simulink model "A2_2_Inverses_Pendel_PR"  (R2023b)
settings: Solver=FixedStepAuto  StartTime=0.0  StopTime=Te  FixedStep=Ts  RelTol=1e-3
values from neighbouring files (symbols this model uses):
  k = lqr(sys, Q, R)    [init_elast_Getriebe.m]    (also in init_inverse_pendel_pr.m)
  params = [ig c s ms CA CM]    [init_DSMS.m]    (also in init_DSMS_vorlage.m = [m c d g]; init_elast_Getriebe.m = [ig c s ms C_A_S C_M_S d]; init_inv.m = [m1 m2 l1 l2 s1 s2 C_1_S g d1 d2 m A_P B_P ig C_M]; init_inverse_pendel.m = [m1 m2 l1 l2 s1 s2 C_1_S g ig C_M_S])
  Ta = 1e-3    (= 0.001)    [init_inverse_pendel_pr.m]
  x1_ic = zeros(4,1)    [init_DSMS.m]    (also in init_DSMS_vorlage.m = zeros(2,1); init_elast_Getriebe.m; init_inv.m; init_inverse_pendel.m)
settings Model: Creator=Flo  LastModifiedBy=Flo

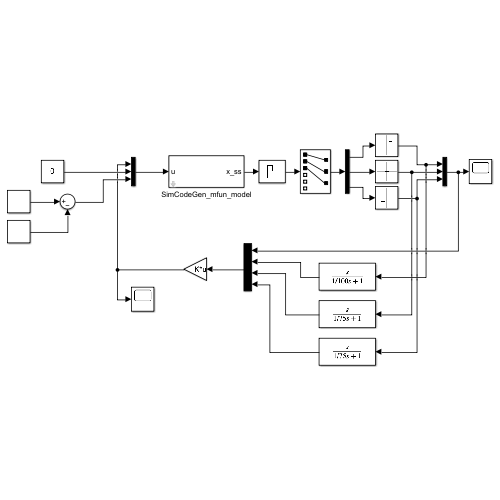
[thumbnail: Simulink's stored preview of the top-level diagram]
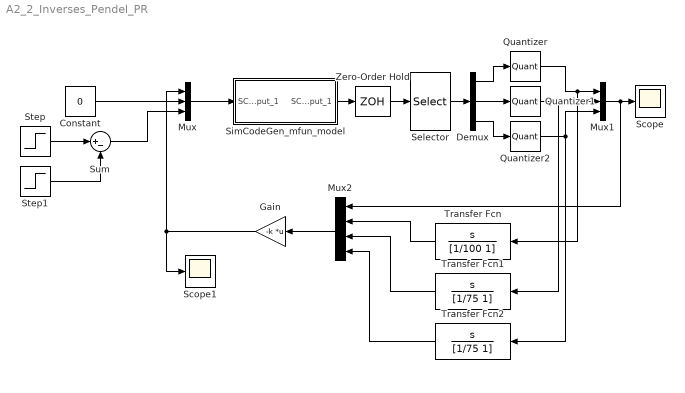
== system A2_2_Inverses_Pendel_PR ==
  Constant : Constant  Value=0
  Demux : Demux  Outputs=3
  Gain : Gain  Gain=-k  Multiplication=Matrix(K*u)
  Mux : Mux  Inputs=3
  Mux1 : Mux  Inputs=3
  Mux2 : Mux
  Quantizer : Quantizer  QuantizationInterval=2*pi/(2048*params(12))
  Quantizer1 : Quantizer  QuantizationInterval=2*pi/4096
  Quantizer2 : Quantizer  QuantizationInterval=2*pi/4096
  Scope : Scope
  Scope1 : Scope
  Selector : Selector  InputPortWidth=6  IndexOptions=Index vector (dialog)  Indices=[1 2 3]  OutputSizes=1
  SimCodeGen_mfun_model : Subsystem  mask{SC_param_0=params, SC_x1_ic=x1_ic}
      mask prompts: SC_param_0 "params"
      mask Display:
      | port_label('input', 1, 'u');
      | port_label('output', 1, 'x_ss');
  Step : Step  SampleTime=0
  Step1 : Step  Time=1.01  SampleTime=0
  Sum : Sum  Inputs=|+-
  Transfer Fcn : TransferFcn  Numerator=[1 0]  Denominator=[1/100 1]
  Transfer Fcn1 : TransferFcn  Numerator=[1 0]  Denominator=[1/75 1]
  Transfer Fcn2 : TransferFcn  Numerator=[1 0]  Denominator=[1/75 1]
  Zero-Order Hold : ZeroOrderHold  SampleTime=Ta
  wires:
  Step/1 -> Sum/1
  Step1/1 -> Sum/2
  Sum/1 -> Mux/3
  Constant/1 -> Mux/2
  Mux/1 -> SimCodeGen_mfun_model/1(SC_input_1)
  SimCodeGen_mfun_model/1(SC_output_1) -> Zero-Order Hold/1
  Gain/1 -> Scope1/1, Mux/1
  Zero-Order Hold/1 -> Selector/1
  Selector/1 -> Demux/1
  Demux/1 -> Quantizer/1
  Demux/2 -> Quantizer1/1
  Demux/3 -> Quantizer2/1
  Mux1/1 -> Mux2/1, Scope/1
  Quantizer2/1 -> Mux1/3, Transfer Fcn2/1
  Quantizer1/1 -> Transfer Fcn1/1, Mux1/2
  Quantizer/1 -> Transfer Fcn/1, Mux1/1
  Mux2/1 -> Gain/1
  Transfer Fcn/1 -> Mux2/2
  Transfer Fcn1/1 -> Mux2/3
  Transfer Fcn2/1 -> Mux2/4

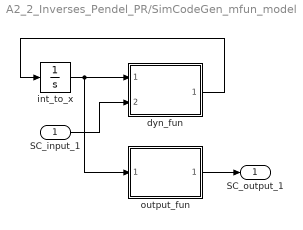
== system A2_2_Inverses_Pendel_PR/SimCodeGen_mfun_model ==
  SC_input_1 : Inport
  dyn_fun : MATLAB Function  TreatAsAtomicUnit=on
  int_to_x : Integrator  InitialCondition=[SC_x1_ic]
  output_fun : MATLAB Function  TreatAsAtomicUnit=on
  SC_output_1 : Outport
  wires:
  int_to_x/1 -> output_fun/1(SC_state), dyn_fun/1(SC_state)
  SC_input_1/1 -> dyn_fun/2(SC_input_0)
  output_fun/1(SC_output_0) -> SC_output_1/1
  dyn_fun/1(SC_state_dot) -> int_to_x/1

== matlab function A2_2_Inverses_Pendel_PR/SimCodeGen_mfun_model/dyn_fun ==
  data: SC_state input size=[6]; SC_state_dot output size=[6]; SC_input_0 input size=[3]; SC_param_0 parameter
function SC_state_dot  = dyn_fun(SC_state, SC_input_0, SC_param_0)
    SC_state_dot = zeros(6, 1);
    SC_state_x_0 = SC_state(1:6);
    SC_eval = zeros(6,1);
    SC_eval(1) = SC_state_x_0(4);
    SC_eval(2) = SC_state_x_0(5);
    SC_eval(3) = SC_state_x_0(6);
    t1 = SC_state_x_0(3);
    t2 = cos(t1);
    t3 = t2 ^ 2;
    t4 = SC_param_0(5);
    t5 = t4 ^ 2;
    t6 = t5 * t3;
    t7 = SC_param_0(6);
    t8 = t7 ^ 2;
    t9 = SC_param_0(18);
    t10 = t9 ^ 2;
    t11 = t10 * t8;
    t12 = t11 * t6;
    t15 = SC_param_0(3);
    t16 = t9 * t15;
    t17 = SC_param_0(9);
    t18 = t17 * t16;
    t21 = t15 ^ 2;
    t22 = t17 ^ 2;
    t23 = t22 * t21;
    t24 = t23 * t6;
    t26 = t8 * t5;
    t27 = SC_param_0(2);
    t28 = t9 * t27;
    t29 = t28 * t26;
    t30 = t16 * t26;
    t32 = SC_param_0(17);
    t33 = t9 * t32;
    t34 = t33 * t26;
    t36 = t10 * t26;
    t38 = t27 * t5;
    t39 = t22 * t15;
    t40 = t39 * t38;
    t41 = t21 * t5;
    t42 = t22 * t41;
    t44 = t15 * t5;
    t45 = t22 * t32;
    t46 = t45 * t44;
    t48 = t22 * t9;
    t49 = t48 * t44;
    t51 = t27 * t8;
    t52 = SC_param_0(8);
    t53 = t52 ^ 2;
    t54 = t53 * t9;
    t55 = t54 * t51;
    t57 = t15 * t27;
    t58 = t22 * t53;
    t59 = t58 * t57;
    t61 = SC_param_0(19);
    t62 = t5 * t61;
    t47 = t32 * t62;
    t73 = -0.24e2 * t18 * t6 * t7 + 0.12e2 * t27 * t53 * t61 + 0.12e2 * t15 * t62 + t27 * t62 + 0.12e2 * t62 * t9 - 0.12e2 * t12 - 0.12e2 * t24 + t29 + 0.12e2 * t30 + 0.12e2 * t34 + 0.12e2 * t36 + t40 + 0.12e2 * t42 + 0.12e2 * t46 + 0.12e2 * t47 + 0.12e2 * t49 + 0.12e2 * t55 + 0.12e2 * t59;
    t74 = SC_state_x_0(2);
    t75 = sin(t74);
    t76 = t75 * t61;
    t77 = sin(t1);
    t78 = cos(t74);
    t79 = t78 * t77;
    t80 = t79 * t76;
    t81 = t5 * t4;
    t82 = t15 * t81;
    t83 = t17 * t9;
    t84 = t83 * t82;
    t87 = t75 ^ 2;
    t88 = t87 * t61;
    t89 = t2 * t4;
    t90 = t89 * t88;
    t92 = t17 * t53 * t57;
    t95 = t5 * t2;
    t96 = t23 * t95;
    t99 = t27 * t81;
    t100 = t17 * t15;
    t101 = t100 * t99;
    t104 = t17 * t32;
    t105 = t104 * t82;
    t108 = t77 * t75;
    t109 = t2 * t78;
    t110 = t109 * t108;
    t111 = t22 ^ 2;
    t116 = t81 * t78;
    t117 = t116 * t108;
    t118 = t15 * t8;
    t119 = t17 * t10;
    t120 = t119 * t118;
    t123 = t2 * t87;
    t124 = t8 * t81;
    t125 = t124 * t123;
    t126 = t83 * t57;
    t129 = SC_param_0(4);
    t130 = t129 ^ 2;
    t131 = t130 * t3;
    t132 = t7 * t5;
    t133 = t132 * t131;
    t136 = t87 * t130;
    t137 = t77 ^ 2;
    t139 = t5 * t137 * t136;
    t140 = t15 * t7;
    t141 = t119 * t140;
    t144 = t21 * t7;
    t145 = t83 * t144;
    t148 = t78 ^ 2;
    t149 = t148 * t130;
    t150 = t6 * t149;
    t91 = t110 * t111;
    t155 = 0.24e2 * t32 * t41 * t91 + 0.2e1 * t101 * t80 + 0.24e2 * t105 * t80 + 0.24e2 * t117 * t120 + 0.2e1 * t125 * t126 - 0.24e2 * t126 * t133 - 0.24e2 * t139 * t141 - 0.24e2 * t139 * t145 + 0.24e2 * t141 * t150 + 0.24e2 * t145 * t150 + 0.24e2 * t80 * t84 + 0.24e2 * t80 * t96 + 0.24e2 * t90 * t92;
    t156 = t3 * t148;
    t157 = t26 * t156;
    t158 = t48 * t57;
    t161 = t7 * t81;
    t162 = t161 * t123;
    t165 = t21 * t8;
    t166 = t83 * t165;
    t169 = t48 * t144;
    t172 = SC_param_0(1);
    t176 = SC_param_0(7) ^ 2;
    t182 = t58 * t16;
    t185 = t27 * t4;
    t186 = t185 * t149;
    t187 = t22 * t52;
    t191 = t3 * t87;
    t192 = t5 ^ 2;
    t195 = t32 * t15;
    t196 = t83 * t195;
    t201 = t21 * t27;
    t206 = t111 * t21;
    t210 = t4 * t130;
    t211 = t210 * t156;
    t212 = t187 * t201;
    t215 = t4 * t78;
    t216 = t215 * t108;
    t217 = t22 * t17;
    t219 = t217 * t53 * t201;
    t197 = t192 * t191;
    t222 = -0.24e2 * t16 * t17 * t172 * t176 * t6 * t7 + 0.24e2 * t110 * t111 * t201 * t53 + 0.2e1 * t110 * t206 * t38 - 0.48e2 * t156 * t182 * t51 - 0.24e2 * t16 * t186 * t187 - 0.24e2 * t196 * t197 * t7 + 0.24e2 * t117 * t166 + 0.24e2 * t117 * t169 - 0.24e2 * t133 * t196 - 0.4e1 * t157 * t158 + 0.2e1 * t158 * t162 + 0.24e2 * t211 * t212 + 0.24e2 * t216 * t219;
    t227 = t27 * t7;
    t228 = t227 * t54;
    t231 = t33 * t161;
    t234 = t16 * t161;
    t237 = t11 * t95;
    t240 = t28 * t161;
    t243 = SC_param_0(13);
    t244 = SC_param_0(12);
    t245 = t244 ^ 2;
    t246 = t245 * t243;
    t247 = t5 * t246;
    t248 = t22 * t57;
    t250 = t3 * t243;
    t251 = t245 * t250;
    t255 = t53 * t15;
    t256 = t22 * t255;
    t259 = t148 * t61;
    t261 = t53 * t28;
    t264 = t3 * t61;
    t268 = t5 * t259;
    t269 = t32 * t8;
    t270 = t9 * t269;
    t273 = t5 * t264;
    t276 = -0.24e2 * t186 * t187 * t195 + 0.12e2 * t246 * t256 * t27 + 0.12e2 * t259 * t261 * t8 + 0.12e2 * t261 * t264 * t8 + 0.24e2 * t228 * t90 + 0.24e2 * t231 * t80 + 0.24e2 * t234 * t80 + 0.24e2 * t237 * t80 + 0.2e1 * t240 * t80 + t247 * t248 - 0.12e2 * t251 * t42 + 0.12e2 * t268 * t270 + 0.12e2 * t270 * t273;
    t277 = t5 * t88;
    t278 = t53 * t57;
    t283 = t3 * t259;
    t286 = t2 * t88;
    t287 = t21 * t81;
    t288 = t17 * t287;
    t297 = t130 * t259;
    t298 = t32 * t44;
    t301 = t75 * t130;
    t303 = t2 * t79 * t301;
    t304 = t15 * t227;
    t305 = t17 * t54;
    t315 = t22 * t54;
    t316 = t315 * t57;
    t325 = t305 * t57;
    t292 = t132 * t18;
    t328 = 0.48e2 * t110 * t316 * t8 + 0.24e2 * t216 * t316 * t7 + 0.24e2 * t216 * t325 * t8 + 0.12e2 * t256 * t259 * t27 + 0.12e2 * t256 * t264 * t27 + 0.4e1 * t27 * t292 * t303 + 0.48e2 * t303 * t304 * t305 + t248 * t268 + t248 * t273 + 0.24e2 * t277 * t278 - 0.24e2 * t283 * t42 + 0.24e2 * t286 * t288 - 0.24e2 * t297 * t298;
    t333 = t52 * t9;
    t334 = t17 * t333;
    t338 = t8 * t4;
    t339 = t10 * t27;
    t351 = t48 * t195;
    t356 = t338 * t149;
    t357 = t32 * t27;
    t365 = t52 * t10 * t51;
    t368 = t8 * t7;
    t369 = t27 * t368;
    t370 = t53 * t10;
    t371 = t370 * t369;
    t374 = t8 ^ 2;
    t375 = t27 * t374;
    t379 = t5 * t245;
    t381 = t83 * t140;
    t384 = t374 * t5;
    t385 = t10 * t32;
    t389 = 0.48e2 * t334 * t57 * t7 * t210 * t156 - 0.24e2 * t52 * t339 * t338 * t303 - 0.24e2 * t21 * t185 * t303 * t187 + 0.24e2 * t196 * t125 + 0.24e2 * t351 * t162 - 0.48e2 * t351 * t157 - 0.24e2 * t333 * t357 * t356 - 0.24e2 * t333 * t57 * t356 + 0.24e2 * t365 * t211 + 0.24e2 * t371 * t216 + 0.24e2 * t370 * t375 * t110 - 0.24e2 * t381 * t379 * t250 + 0.24e2 * t385 * t384 * t110;
    t393 = t10 * t15;
    t401 = t22 * t10;
    t402 = t401 * t140;
    t405 = t5 * t109;
    t406 = t405 * t108;
    t407 = t22 * t33;
    t411 = t22 * t16;
    t415 = t79 * t301;
    t416 = t22 * t201;
    t420 = t27 * t2;
    t421 = t53 * t21;
    t422 = t22 * t421;
    t426 = t10 * t51;
    t430 = t8 * t2;
    t431 = t53 * t339;
    t435 = t22 * t393;
    t436 = t435 * t26;
    t439 = t3 * t2;
    t441 = t439 * t78 * t108;
    t444 = t3 * t78;
    t445 = t444 * t108;
    t446 = t17 * t393;
    t450 = 0.2e1 * t110 * t339 * t384 + 0.24e2 * t110 * t384 * t393 + 0.48e2 * t118 * t406 * t407 - 0.72e2 * t124 * t445 * t446 + 0.4e1 * t406 * t411 * t51 + 0.24e2 * t41 * t9 * t91 + 0.2e1 * t415 * t416 * t95 + 0.24e2 * t415 * t420 * t422 + 0.2e1 * t415 * t426 * t95 + 0.24e2 * t415 * t430 * t431 + 0.48e2 * t110 * t436 + 0.24e2 * t117 * t402 - 0.24e2 * t436 * t441;
    t452 = t9 * t21;
    t453 = t22 * t452;
    t454 = t453 * t26;
    t464 = t217 * t452;
    t476 = t18 * t227;
    t484 = t7 * t4;
    t437 = t3 * t149;
    t438 = t325 * t7;
    t495 = -0.48e2 * t368 * t441 * t446 * t5 + 0.2e1 * t117 * t18 * t51 + 0.2e1 * t117 * t227 * t411 + 0.24e2 * t123 * t316 * t484 + 0.24e2 * t123 * t325 * t338 - 0.24e2 * t132 * t191 * t325 - 0.48e2 * t132 * t441 * t464 - 0.72e2 * t161 * t445 * t453 + 0.48e2 * t110 * t454 - 0.2e1 * t139 * t476 - 0.2e1 * t150 * t476 - 0.24e2 * t437 * t438 - 0.24e2 * t441 * t454;
    t500 = t17 * t33;
    t507 = t500 * t140;
    t515 = t17 * t255;
    t522 = t22 * t195;
    t526 = t9 * t51;
    t530 = t9 * t118;
    t486 = t137 * t136;
    t543 = 0.24e2 * t117 * t118 * t500 + 0.24e2 * t117 * t140 * t407 + 0.24e2 * t185 * t515 * t80 + 0.2e1 * t248 * t80 * t95 + 0.24e2 * t256 * t420 * t80 + 0.24e2 * t261 * t430 * t80 + 0.24e2 * t261 * t484 * t80 + 0.24e2 * t411 * t80 * t95 + 0.24e2 * t522 * t80 * t95 + 0.2e1 * t526 * t80 * t95 + 0.24e2 * t530 * t80 * t95 - 0.24e2 * t139 * t507 + 0.24e2 * t150 * t507 - 0.24e2 * t438 * t486;
    t550 = SC_param_0(10);
    t551 = t550 * t61;
    t552 = t9 * t5;
    t558 = t130 * t61;
    t559 = t10 * t5;
    t562 = t32 * t5;
    t565 = t32 ^ 2;
    t569 = t565 * t5;
    t572 = t27 * t53;
    t578 = t27 ^ 2;
    t579 = t53 * t578;
    t582 = t53 ^ 2;
    t588 = 0.12e2 * t10 * t192 * t88 + 0.12e2 * t192 * t565 * t88 + 0.24e2 * t270 * t80 * t95 + 0.12e2 * t578 * t582 * t88 + t38 * t551 + 0.12e2 * t41 * t558 + 0.12e2 * t44 * t551 + 0.12e2 * t551 * t552 + 0.12e2 * t551 * t562 + 0.12e2 * t551 * t572 + 0.12e2 * t558 * t559 + 0.12e2 * t558 * t569 + 0.12e2 * t558 * t579;
    t589 = t578 * t5;
    t594 = t5 * t550;
    t597 = t192 * t87;
    t598 = t10 * t9;
    t599 = t598 * t8;
    t602 = t5 * t148;
    t603 = t598 * t374;
    t608 = t3 ^ 2;
    t609 = t5 * t608;
    t612 = t5 * t130;
    t617 = t21 * t15;
    t618 = t22 * t617;
    t621 = t111 * t617;
    t628 = 0.12e2 * t192 * t21 * t88 + 0.12e2 * t11 * t594 + 0.12e2 * t23 * t594 + t558 * t589 + 0.12e2 * t597 * t599 + 0.12e2 * t597 * t618 + 0.12e2 * t599 * t612 + 0.12e2 * t6 * t603 + 0.12e2 * t602 * t603 + 0.12e2 * t602 * t621 - 0.12e2 * t603 * t609 - 0.12e2 * t609 * t621 + 0.12e2 * t612 * t618;
    t632 = t78 * t108;
    t633 = t130 * t2;
    t634 = t4 * t633;
    t639 = t8 * t602;
    t642 = t8 * t6;
    t645 = t5 * t87;
    t646 = t27 * t645;
    t650 = t486;
    t651 = t45 * t41;
    t654 = t437;
    t661 = t58 * t201;
    t666 = t4 * t149;
    t669 = t4 * t123;
    t672 = t5 * t191;
    t675 = 0.24e2 * t217 * t287 * t32 * t632 - 0.48e2 * t304 * t334 * t632 * t634 + 0.24e2 * t195 * t58 * t646 + 0.2e1 * t158 * t639 + 0.2e1 * t158 * t642 - 0.24e2 * t212 * t666 + 0.24e2 * t219 * t669 + 0.12e2 * t6 * t621 - 0.12e2 * t650 * t651 - 0.12e2 * t650 * t661 + 0.12e2 * t651 * t654 - 0.12e2 * t654 * t661 - 0.12e2 * t661 * t672;
    t676 = t23 * t38;
    t679 = t217 * t21;
    t691 = t5 * t439;
    t695 = t5 * t156;
    t696 = t15 * t368;
    t697 = t119 * t696;
    t700 = t217 * t9;
    t701 = t700 * t144;
    t704 = t393 * t26;
    t709 = t368 * t81;
    t713 = t339 * t26;
    t657 = t217 * t617;
    t658 = t632 * t81 * t3;
    t670 = t632 * t621;
    t719 = 0.2e1 * t339 * t632 * t709 + 0.24e2 * t393 * t632 * t709 + 0.2e1 * t632 * t679 * t99 - t650 * t676 - 0.12e2 * t650 * t704 - t650 * t713 - t654 * t676 + 0.12e2 * t654 * t704 - t654 * t713 - 0.24e2 * t657 * t658 - 0.24e2 * t670 * t691 + 0.24e2 * t670 * t95 - 0.24e2 * t695 * t697 - 0.24e2 * t695 * t701;
    t732 = t8 * t645;
    t736 = t5 * t149;
    t743 = t385 * t26;
    t754 = t3 * t550;
    t758 = t370 * t51;
    t720 = t632 * t603;
    t761 = -0.24e2 * t118 * t33 * t736 + 0.24e2 * t357 * t54 * t732 - 0.24e2 * t368 * t598 * t658 - 0.24e2 * t381 * t5 * t754 + 0.24e2 * t385 * t632 * t709 + 0.24e2 * t351 * t639 + 0.24e2 * t351 * t642 - 0.24e2 * t351 * t736 - 0.12e2 * t650 * t743 + 0.12e2 * t654 * t743 - 0.12e2 * t654 * t758 - 0.24e2 * t691 * t720 + 0.24e2 * t720 * t95;
    t775 = t8 * t148;
    t779 = t8 * t3;
    t783 = t48 * t41;
    t791 = t5 * t131;
    t739 = t27 * t182;
    t796 = 0.24e2 * t287 * t632 * t700 + 0.24e2 * t54 * t57 * t732 - 0.24e2 * t141 * t791 - 0.24e2 * t145 * t791 + 0.24e2 * t182 * t646 - 0.24e2 * t365 * t666 + 0.24e2 * t371 * t669 - 0.12e2 * t650 * t758 - 0.12e2 * t650 * t783 + 0.12e2 * t654 * t783 - 0.12e2 * t672 * t758 + 0.24e2 * t739 * t775 + 0.24e2 * t739 * t779;
    t798 = t77 * t76;
    t799 = t10 * t7;
    t772 = t185 * t297;
    t777 = t798 * t116;
    t830 = -0.24e2 * t32 * t52 * t772 + 0.24e2 * t231 * t286 + 0.24e2 * t234 * t286 + 0.2e1 * t240 * t286 - 0.2e1 * t283 * t29 - 0.24e2 * t283 * t30 - 0.24e2 * t283 * t34 - 0.24e2 * t283 * t46 - 0.24e2 * t283 * t49 - 0.24e2 * t283 * t55 + 0.24e2 * t286 * t84 - 0.24e2 * t333 * t772 + 0.24e2 * t777 * t799;
    t833 = t52 * t15;
    t839 = t17 * t21;
    t847 = t48 * t165;
    t850 = t81 * t123;
    t853 = t401 * t118;
    t858 = t608 * t148;
    t859 = t5 * t858;
    t862 = t439 * t87;
    t863 = t81 * t862;
    t870 = 0.2e1 * t101 * t286 + 0.24e2 * t105 * t286 + 0.24e2 * t120 * t850 - 0.72e2 * t120 * t863 + 0.24e2 * t166 * t850 - 0.2e1 * t283 * t40 - 0.24e2 * t283 * t59 + 0.24e2 * t402 * t850 - 0.60e2 * t695 * t847 - 0.60e2 * t695 * t853 - 0.24e2 * t772 * t833 + 0.24e2 * t777 * t839 + 0.24e2 * t847 * t859 + 0.24e2 * t853 * t859;
    t883 = t197;
    t889 = t10 * t32 * t374;
    t895 = t9 * t565 * t8;
    t898 = t10 * t269;
    t904 = t176 * t10 * t172;
    t907 = t8 * t130;
    t908 = t9 * t578;
    t909 = t53 * t908;
    t912 = -0.24e2 * t141 * t883 - 0.24e2 * t145 * t883 + 0.24e2 * t169 * t850 - 0.72e2 * t169 * t863 + 0.12e2 * t26 * t904 + 0.12e2 * t270 * t594 + 0.12e2 * t6 * t889 + 0.12e2 * t602 * t889 + 0.12e2 * t612 * t895 + 0.24e2 * t612 * t898 + 0.48e2 * t697 * t859 + 0.48e2 * t701 * t859 + 0.12e2 * t907 * t909;
    t915 = t8 * t87;
    t919 = t374 * t148;
    t922 = t374 * t3;
    t933 = t111 * t452;
    t943 = 0.12e2 * t582 * t908 * t915 - 0.12e2 * t36 * t754 + 0.12e2 * t431 * t907 + 0.12e2 * t431 * t919 + 0.12e2 * t431 * t922 + 0.12e2 * t435 * t597 + 0.12e2 * t435 * t612 + 0.24e2 * t453 * t597 + 0.24e2 * t453 * t612 + t526 * t594 + 0.12e2 * t530 * t594 + 0.12e2 * t6 * t933 + 0.12e2 * t602 * t933;
    t945 = t8 * t550;
    t952 = t598 * t384;
    t955 = t598 * t709;
    t966 = t9 * t165;
    t969 = t10 * t118;
    t977 = t598 * t26;
    t913 = t578 * t612;
    t914 = t8 * t9;
    t980 = 0.24e2 * t123 * t955 - 0.12e2 * t131 * t977 - 0.36e2 * t156 * t952 + 0.12e2 * t246 * t36 + 0.12e2 * t261 * t945 + 0.12e2 * t411 * t594 + 0.13e2 * t426 * t612 - 0.12e2 * t599 * t883 + 0.12e2 * t612 * t966 + 0.24e2 * t612 * t969 + 0.24e2 * t858 * t952 - 0.24e2 * t862 * t955 + t913 * t914;
    t988 = t10 * t15 * t374;
    t994 = t10 * t375;
    t1001 = t32 * t21;
    t1002 = t22 * t1001;
    t1006 = t22 * t565 * t15;
    t1011 = 0.24e2 * t1002 * t597 + 0.24e2 * t1002 * t612 + 0.12e2 * t1006 * t612 - 0.12e2 * t149 * t977 + t426 * t597 + 0.12e2 * t597 * t895 + 0.24e2 * t597 * t898 + 0.12e2 * t597 * t966 + 0.24e2 * t597 * t969 + 0.12e2 * t6 * t988 + t6 * t994 + 0.12e2 * t602 * t988 + t602 * t994;
    t1016 = t111 * t1001;
    t1024 = t176 * t9 * t172;
    t1029 = t243 * t61;
    t1033 = t21 * t612;
    t1042 = t10 * t612;
    t1045 = t9 * t44;
    t1048 = t15 * t192;
    t1052 = 0.12e2 * t1029 * t379 * t9 + 0.24e2 * t1048 * t88 * t9 + 0.13e2 * t15 * t38 * t558 + 0.13e2 * t38 * t558 * t9 + 0.12e2 * t1006 * t597 + 0.12e2 * t1016 * t6 + 0.12e2 * t1016 * t602 + 0.12e2 * t1024 * t62 - 0.12e2 * t1033 * t259 - 0.12e2 * t1042 * t259 + 0.24e2 * t1045 * t558 + 0.12e2 * t261 * t558 + 0.12e2 * t522 * t594;
    t1053 = t27 * t192;
    t1064 = t9 * t562;
    t1072 = t565 * t612;
    t1086 = t53 * t357;
    t1089 = 0.24e2 * t192 * t32 * t88 * t9 + 0.24e2 * t1048 * t32 * t88 + t1053 * t15 * t88 + t1053 * t32 * t88 + t1053 * t88 * t9 + 0.12e2 * t172 * t176 * t47 + 0.13e2 * t32 * t38 * t558 + 0.24e2 * t1064 * t558 - 0.12e2 * t1072 * t259 + 0.12e2 * t1086 * t558 + 0.12e2 * t259 * t36 + 0.12e2 * t264 * t36 + 0.24e2 * t298 * t558;
    t1094 = t15 * t172;
    t1098 = t27 * t172;
    t1101 = t578 * t130;
    t1102 = t53 * t1101;
    t1109 = t172 * t61;
    t1110 = t176 * t27;
    t1127 = t617 * t5;
    t1128 = t22 * t1127;
    t1050 = t245 * t1029;
    t1131 = 0.12e2 * t1029 * t15 * t379 + t1029 * t27 * t379 + 0.12e2 * t1029 * t32 * t379 + 0.12e2 * t1094 * t176 * t62 + t1098 * t176 * t62 + 0.12e2 * t1109 * t1110 * t53 + t53 * t589 * t88 + 0.12e2 * t1050 * t572 - 0.12e2 * t1102 * t259 - 0.12e2 * t1128 * t131 + 0.12e2 * t259 * t42 + 0.12e2 * t264 * t42 + 0.12e2 * t278 * t558;
    t1140 = t111 * t201;
    t1154 = t81 * t657;
    t1085 = t176 * t22;
    t1159 = t21 * t1085;
    t1162 = t172 * t5;
    t1164 = t176 * t15;
    t1087 = t1162 * t1164;
    t1170 = t1087 * t22 * t27 - 0.12e2 * t1159 * t172 * t6 - 0.12e2 * t149 * t256 * t578 + 0.2e1 * t201 * t217 * t850 - 0.12e2 * t1128 * t149 - 0.12e2 * t1128 * t650 + 0.12e2 * t1128 * t654 + t1140 * t602 - 0.2e1 * t1140 * t695 + 0.24e2 * t1154 * t632 + t39 * t913 + t416 * t597 + 0.13e2 * t416 * t612 - 0.12e2 * t416 * t791;
    t1183 = t27 * t156;
    t1184 = t111 * t421;
    t1123 = t1098 * t53 * t176;
    t1203 = t256 * t578 * t645 - 0.24e2 * t1045 * t297 - 0.24e2 * t1064 * t297 + 0.24e2 * t1086 * t277 + 0.12e2 * t1123 * t39 - 0.24e2 * t1183 * t1184 + 0.12e2 * t268 * t411 + 0.12e2 * t268 * t522 + t268 * t526 + 0.12e2 * t273 * t411 + 0.12e2 * t273 * t522 + t273 * t526 + 0.24e2 * t422 * t646;
    t1206 = t10 * t161;
    t1228 = t8 * t612;
    t1229 = t9 * t57;
    t1234 = 0.2e1 * t10 * t369 * t850 + 0.24e2 * t1206 * t286 + 0.13e2 * t1228 * t1229 + 0.12e2 * t247 * t270 + 0.24e2 * t261 * t277 + 0.12e2 * t268 * t530 + 0.12e2 * t273 * t530 - 0.24e2 * t283 * t36 - 0.12e2 * t426 * t791 - 0.12e2 * t650 * t977 + 0.12e2 * t654 * t977 - 0.2e1 * t695 * t994 - 0.12e2 * t736 * t966;
    t1242 = t8 * t597;
    t1253 = t172 * t26;
    t1265 = t27 * t907;
    t1193 = t176 * t1253;
    t1269 = 0.24e2 * t10 * t696 * t850 + 0.12e2 * t1253 * t16 * t176 + 0.12e2 * t1265 * t16 * t53 - 0.12e2 * t149 * t8 * t909 - 0.24e2 * t156 * t374 * t431 + t1193 * t28 + t1229 * t1242 + 0.24e2 * t632 * t955 - 0.12e2 * t642 * t904 - 0.24e2 * t695 * t988 - 0.24e2 * t736 * t969 - 0.12e2 * t791 * t969 - 0.12e2 * t883 * t969;
    t1275 = t176 * t9;
    t1279 = t27 * t612;
    t1296 = t9 * t195;
    t1222 = t1275 * t172 * t8;
    t1232 = t407 * t15;
    t1308 = 0.12e2 * t1265 * t33 * t53 + 0.24e2 * t368 * t385 * t850 + 0.12e2 * t1193 * t33 + 0.12e2 * t1222 * t572 + 0.24e2 * t1232 * t612 + 0.24e2 * t1242 * t1296 + 0.13e2 * t1279 * t411 + 0.24e2 * t431 * t732 - 0.12e2 * t435 * t736 - 0.24e2 * t453 * t736 - 0.12e2 * t453 * t791 - 0.24e2 * t695 * t889 + t732 * t909 - 0.12e2 * t883 * t898;
    t1311 = t9 * t357;
    t1330 = t27 * t597;
    t1339 = 0.24e2 * t1001 * t217 * t850 - 0.24e2 * t1002 * t736 - 0.12e2 * t1002 * t791 - 0.12e2 * t1002 * t883 - 0.12e2 * t1006 * t736 - 0.24e2 * t1016 * t695 + 0.24e2 * t1228 * t1296 + 0.13e2 * t1228 * t1311 + 0.13e2 * t1279 * t522 + t1330 * t522 - 0.12e2 * t736 * t895 - 0.24e2 * t736 * t898 - 0.12e2 * t791 * t898;
    t1340 = t15 * t1162;
    t1341 = t176 * t32;
    t1345 = t27 * t130;
    t1346 = t15 * t1345;
    t1347 = t53 * t32;
    t1375 = 0.12e2 * t1340 * t1341 * t22 + 0.12e2 * t1346 * t1347 * t22 - 0.24e2 * t368 * t446 * t609 - 0.24e2 * t464 * t609 * t7 + 0.24e2 * t1232 * t597 + t1330 * t411 + 0.12e2 * t247 * t522 + 0.24e2 * t435 * t639 + 0.24e2 * t453 * t639 + 0.24e2 * t453 * t642 - 0.12e2 * t453 * t883 + 0.24e2 * t464 * t850 - 0.24e2 * t695 * t933;
    t1379 = t8 * t609;
    t1401 = t111 * t1127;
    t1404 = 0.12e2 * t1275 * t1340 * t22 + 0.12e2 * t246 * t261 * t8 + t1140 * t6 + t1242 * t1311 + 0.12e2 * t1346 * t315 - 0.12e2 * t1379 * t435 - 0.12e2 * t1379 * t453 + 0.24e2 * t1401 * t858 + 0.12e2 * t247 * t411 + t247 * t526 + 0.12e2 * t247 * t530 - 0.12e2 * t251 * t36 + 0.24e2 * t435 * t642;
    t1421 = t578 * t87;
    t1426 = t27 * t148;
    t1429 = t27 * t3;
    t1435 = t27 * t550;
    t1440 = 0.12e2 * t1421 * t15 * t22 * t582 + 0.12e2 * t1101 * t256 + 0.24e2 * t1154 * t123 - 0.24e2 * t1154 * t862 + 0.12e2 * t1159 * t1162 + 0.12e2 * t1184 * t1426 + 0.12e2 * t1184 * t1429 + 0.12e2 * t1345 * t422 - 0.36e2 * t1401 * t156 + 0.12e2 * t1435 * t256 + 0.12e2 * t246 * t42 + t248 * t594 - 0.12e2 * t42 * t754 - 0.12e2 * t618 * t883;
    t1381 = t328 + t543 + t1339 + t1308 + t450 + t495 + t276 + t943 + t980 + t1011 + t1052 + t1089 + t1131 + t1170 + t1203 + t1234;
    t1382 = t1269 + t222 + t588 + t628 + t1440 + t1404 + t1375 + t389 + t155 + t870 + t912 + t675 + t719 + t761 + t796 + t830;
    t1446 = 0.1e1 / (t1382 + t1381);
    t1448 = SC_input_0(3);
    t1449 = t129 * t1448;
    t1451 = SC_state_x_0(1);
    t1452 = sin(t1451);
    t1454 = SC_input_0(2);
    t1458 = cos(t1451);
    t1459 = t1454 * t1458;
    t1384 = SC_eval(2);
    t1385 = SC_eval(3);
    t1463 = t1384 + t1385;
    t1464 = t914;
    t1465 = t39 + t1464;
    t1466 = t1465 * t1463;
    t1468 = t1384 * t4;
    t1469 = t9 * t7;
    t1470 = t100 + t1469;
    t1478 = t1470 * t4;
    t1497 = t1463 ^ 2;
    t1498 = t1470 * t1497;
    t1509 = t1384 ^ 2;
    t1510 = t27 * t52;
    t1511 = t4 * t15;
    t1512 = t32 * t4;
    t1513 = t9 * t4;
    t1519 = t77 * t2;
    t1522 = t77 * t1470;
    t1398 = SC_eval(1);
    t1528 = t1449 * t109 + t4 * t1454 * t1452 * t75 - t1449 * t108 + t129 * t1459 + t244 * SC_input_0(1) - 0.4e1 * t1398 * (t1466 * t2 + t1468 * t1470) * t148 * t77 - (0.4e1 * t1398 * (t3 * t1466 + t1478 * (t1384 + t1385 / 0.2e1) * t2 + (t9 * (t5 - t8) + t15 * (t5 - t22) + t572 + t562) * t1384 / 0.2e1 - t1385 * t1465 / 0.2e1) * t75 + t1498 * t77 * t129) * t78 + 0.2e1 * t1398 * t1470 * t4 * t1385 * t77 * t87 - t75 * (t2 * t1498 + (t1510 + t1511 + t1512 + t1513) * t1509) * t129 - t1398 * (-0.2e1 * t1466 * t1519 - 0.2e1 * t1468 * t1522 + SC_param_0(14));
    t1530 = t2 * t108;
    t1531 = t10 * t338;
    t1532 = t1531 * t1530;
    t1534 = t381 * t89 * t108;
    t1536 = t21 * t4;
    t1537 = t22 * t1536;
    t1538 = t1537 * t1530;
    t1539 = t1531 * t444;
    t1541 = t381 * t4 * t444;
    t1543 = t1537 * t444;
    t1544 = t530 * t215;
    t1545 = t270 * t215;
    t1546 = t11 * t215;
    t1547 = t23 * t215;
    t1548 = t522 * t215;
    t1549 = t411 * t215;
    t1551 = t52 * t28;
    t1552 = t1551 * t8 * t78;
    t1555 = t22 * t833 * t27 * t78;
    t1556 = t78 * t61;
    t1557 = t1511 * t1556;
    t1558 = t1512 * t1556;
    t1559 = t1513 * t1556;
    t1560 = t1510 * t1556;
    t1561 = t1532 + 0.2e1 * t1534 + t1538 - t1539 - 0.2e1 * t1541 - t1543 + t1544 + t1545 + t1546 + t1547 + t1548 + t1549 + t1552 + t1555 + t1557 + t1558 + t1559 + t1560;
    t1562 = t1561 * t129;
    t1569 = t1398 ^ 2;
    t1577 = t32 + t9 + t15;
    t1582 = SC_param_0(11);
    t1583 = t1470 * t1582;
    t1584 = t77 * t1583;
    t1592 = t1465 * t1569;
    t1596 = t1385 ^ 2;
    t1604 = -t215 * t1459 - (t89 + t7) * t1448 + 0.2e1 * t148 * t1569 * t77 * (t1465 * t2 + t1478) - t78 * (-t75 * (0.2e1 * t1465 * t3 + 0.2e1 * t1478 * t2 + t1577 * t5 - t1464 - t39 + t572) * t1569 - t1584) + t75 * (t1470 * t2 + t1577 * t4 + t1510) * t1582 - t77 * (t2 * t1592 + t4 * (-0.2e1 * t1384 * t1385 + t1569 - t1596) * t1470) - SC_param_0(15) * t1384;
    t1612 = t5 * t108;
    t1614 = t9 * t32 * t7;
    t1617 = t9 * t227;
    t1620 = t9 * t140;
    t1631 = t17 * t195;
    t1634 = t17 * t57;
    t1644 = 0.12e2 * t108 * t261 * t7 + 0.12e2 * t108 * t27 * t515 - 0.12e2 * t109 * t261 * t7 - 0.12e2 * t109 * t27 * t515 + 0.12e2 * t1612 * t1614 + t1612 * t1617 + 0.12e2 * t1612 * t1620 + 0.12e2 * t1612 * t1631 + t1612 * t1634 + 0.12e2 * t1612 * t18 - t1617 * t405 - t1634 * t405 + 0.12e2 * t1532 + 0.24e2 * t1534 + 0.12e2 * t1538 - 0.24e2 * t1541 + 0.12e2 * t1546;
    t1645 = t4 * t109;
    t1646 = t333 * t227;
    t1649 = t17 * t52 * t57;
    t1655 = t10 * t108 * t132 + t108 * t17 * t41 + t1645 * t1646 + t1645 * t1649 - t1539 - t1543 + t1544 + t1545 + t1547 + t1548 + t1549 + t1552 + t1555 + t1557 + t1558 + t1559 + t1560;
    t1658 = (t1644 + 0.12e2 * t1655) * t129;
    t1597 = t1465 * t75 * t1569;
    t1685 = -t7 * t1448 + 0.2e1 * t148 * t1592 * t1519 - (-t1470 * t1569 * t2 * t4 * t75 - 0.2e1 * t1597 * t3 - t1584 + t1597) * t78 - t2 * (-t1583 * t75 + t1592 * t77) - t87 * t1522 * t4 * t1569 - t1522 * t4 * t1509 - SC_param_0(16) * t1385;
    SC_eval(4) = t1446 * t1528 * t73 + 0.12e2 * t1446 * t1562 * t1604 - t1446 * t1658 * t1685;
    t1688 = t1528 * t1446;
    t1690 = t8 * t156;
    t1691 = t411 * t1690;
    t1692 = 0.4e1 * t1691;
    t1625 = t10 * t374;
    t1626 = t2 * t632;
    t1695 = t1626 * t1625;
    t1696 = 0.2e1 * t1695;
    t1698 = t10 * t368 * t4;
    t1699 = t1698 * t632;
    t1700 = 0.2e1 * t1699;
    t1703 = t1626 * t206;
    t1704 = 0.2e1 * t1703;
    t1705 = t217 * t1536;
    t1706 = t1705 * t632;
    t1707 = 0.2e1 * t1706;
    t1708 = t9 * t484;
    t1709 = t1708 * t286;
    t1710 = 0.2e1 * t1709;
    t1711 = t17 * t1511;
    t1712 = t1711 * t286;
    t1713 = 0.2e1 * t1712;
    t1716 = t18 * t7 * t130 * t110;
    t1717 = 0.4e1 * t1716;
    t1719 = t22 * t21 * t130;
    t1632 = t111 * t21;
    t1721 = t148 * t1632;
    t1723 = t3 * t1632;
    t1725 = t22 * t15 * t550;
    t1726 = t10 * t907;
    t1727 = t10 * t919;
    t1728 = t10 * t922;
    t1729 = t9 * t945;
    t1730 = t176 * t1109;
    t1731 = t551 - t1692 + t1696 + t1700 + t1704 + t1707 + t1710 + t1713 + t1717 + t1719 + t1721 + t1723 + t1725 + t1726 + t1727 + t1728 + t1729 + t1730;
    t1732 = t1050;
    t1733 = t32 * t558;
    t1734 = t9 * t558;
    t1735 = t27 * t558;
    t1736 = t15 * t558;
    t1737 = t1726 * t156;
    t1738 = t137 * t87;
    t1739 = t1726 * t1738;
    t1740 = t1698 * t123;
    t1741 = 0.2e1 * t1740;
    t1742 = t530 * t645;
    t1743 = t270 * t645;
    t1744 = t261 * t915;
    t1745 = t411 * t645;
    t1746 = t411 * t775;
    t1747 = 0.2e1 * t1746;
    t1748 = t411 * t779;
    t1749 = 0.2e1 * t1748;
    t1750 = t522 * t645;
    t1752 = t9 * t779 * t259;
    t1753 = 0.2e1 * t1752;
    t1756 = t283 * t39;
    t1757 = 0.2e1 * t1756;
    t1758 = t1719 * t156;
    t1759 = t1719 * t1738;
    t1760 = t1732 + t1733 + t1734 + t1735 + t1736 - t1737 - t1739 + t1741 + t1742 + t1743 + t1744 + t1745 + t1747 + t1749 + t1750 - t1753 - t1757 - t1758 - t1759;
    t1762 = t1705 * t123;
    t1763 = 0.2e1 * t1762;
    t1765 = t256 * t27 * t87;
    t1766 = t1464 * t259;
    t1767 = t1464 * t264;
    t1768 = t552 * t88;
    t1769 = t562 * t88;
    t1770 = t39 * t259;
    t1771 = t39 * t264;
    t1772 = t572 * t88;
    t1773 = t44 * t88;
    t1774 = t1464 * t246;
    t1775 = t33 * t907;
    t1776 = t15 * t130;
    t1777 = t48 * t1776;
    t1778 = t1222;
    t1780 = t156 * t1625;
    t1781 = 0.2e1 * t1780;
    t1782 = t11 * t645;
    t1783 = t16 * t907;
    t1784 = t28 * t907;
    t1785 = t1763 + t1765 + t1766 + t1767 + t1768 + t1769 + t1770 + t1771 + t1772 + t1773 + t1774 + t1775 + t1777 + t1778 - t1781 + t1782 + t1783 + t1784;
    t1786 = t39 * t246;
    t1787 = t45 * t1776;
    t1789 = t1094 * t1085;
    t1790 = t23 * t645;
    t1791 = t39 * t1345;
    t1792 = t206 * t156;
    t1793 = 0.2e1 * t1792;
    t1794 = t83 * t118;
    t1795 = t1794 * t216;
    t1796 = 0.2e1 * t1795;
    t1797 = t48 * t140;
    t1798 = t1797 * t216;
    t1799 = 0.2e1 * t1798;
    t1801 = t48 * t118 * t110;
    t1802 = 0.4e1 * t1801;
    t1804 = t23 * t633 * t632;
    t1805 = 0.2e1 * t1804;
    t1807 = t100 * t215 * t798;
    t1808 = 0.2e1 * t1807;
    t1810 = t39 * t109 * t798;
    t1811 = 0.2e1 * t1810;
    t1813 = t1464 * t109 * t798;
    t1814 = 0.2e1 * t1813;
    t1816 = t1469 * t215 * t798;
    t1817 = 0.2e1 * t1816;
    t1818 = t381 * t654;
    t1819 = 0.2e1 * t1818;
    t1820 = t381 * t650;
    t1821 = 0.2e1 * t1820;
    t1822 = t1794 * t669;
    t1823 = 0.2e1 * t1822;
    t1824 = t1797 * t669;
    t1825 = 0.2e1 * t1824;
    t1827 = t11 * t633 * t632;
    t1828 = 0.2e1 * t1827;
    t1829 = t1786 + t1787 + t1789 + t1790 + t1791 - t1793 + t1796 + t1799 + t1802 + t1805 + t1808 + t1811 + t1814 + t1817 - t1819 - t1821 + t1823 + t1825 + t1828;
    t1834 = t2 * t148;
    t1835 = t130 * t1834;
    t1836 = t104 * t1511;
    t1837 = t1836 * t1835;
    t1838 = t1631 * t850;
    t1839 = t1631 * t634;
    t1840 = t1614 * t850;
    t1841 = t1614 * t634;
    t1842 = t18 * t850;
    t1843 = t18 * t634;
    t1844 = t4 * t439;
    t1846 = t18 * t8 * t1844;
    t1848 = t411 * t7 * t1844;
    t1849 = t1620 * t850;
    t1850 = t10 * t484;
    t1851 = t1850 * t1835;
    t1852 = t1620 * t634;
    t1853 = t1617 * t634;
    t1855 = t1024 * t7 * t89;
    t1857 = t245 * t2 * t243;
    t1858 = t1708 * t1857;
    t1859 = -t1837 + t551 + t1838 + t1839 + t1840 + t1841 + t1842 + t1843 + t1846 + t1848 + t1849 - t1851 + t1852 + t1853 + t1855 + t1858;
    t1860 = t17 * t1536;
    t1861 = t1860 * t1835;
    t1862 = t1634 * t634;
    t1865 = t17 * t1164 * t172 * t89;
    t1866 = t1711 * t1857;
    t1867 = t1649 * t1835;
    t1868 = t92 * t669;
    t1870 = t839 * t210 * t632;
    t1871 = t96 * t632;
    t1873 = t4 * t3;
    t1875 = t679 * t1873 * t632;
    t1877 = t83 * t1511;
    t1878 = t1877 * t1835;
    t1879 = -t1861 + t1862 + t1865 + t1866 - t1692 + t1696 + t1700 + t1704 + t1707 + t1710 + t1713 - t1867 + t1868 + t1870 + 0.2e1 * t1871 + 0.2e1 * t1875 - t1878;
    t1881 = t4 * t1834;
    t1882 = t1794 * t1881;
    t1883 = t1797 * t1881;
    t1884 = t439 * t148;
    t1885 = t4 * t1884;
    t1886 = t1794 * t1885;
    t1888 = t1797 * t1885;
    t1890 = t381 * t672;
    t1892 = t33 * t484;
    t1893 = t1892 * t1835;
    t1894 = t1646 * t1835;
    t1895 = t228 * t669;
    t1897 = t799 * t210 * t632;
    t1898 = t16 * t484;
    t1899 = t1898 * t1835;
    t1900 = t237 * t632;
    t1902 = t10 * t368;
    t1904 = t1902 * t1873 * t632;
    t1907 = t18 * t338 * t445;
    t1910 = t411 * t484 * t445;
    t1913 = t110 * t292;
    t1915 = t1882 + t1883 - 0.2e1 * t1886 - 0.2e1 * t1888 + 0.4e1 * t1890 - t1893 - t1894 + t1895 + t1897 - t1899 + 0.2e1 * t1900 + 0.2e1 * t1904 + t1717 + 0.2e1 * t1907 + 0.2e1 * t1910 + 0.4e1 * t1913 + t1719;
    t1916 = t1721 + t1723 + t1725 + t1726 + t1727 + t1728 + t1729 + t1730 + t1732 + t1733 + t1734 + t1735 + t1736 - t1737 - t1739 + t1741 + t1742;
    t1919 = t1743 + t1744 + t1745 + t1747 + t1749 + t1750 - t1753 - t1757 - t1758 - t1759 + t1763 + t1765 + t1766 + t1767 + t1768 + t1769;
    t1920 = t1770 + t1771 + t1772 + t1773 + t1774 + t1775 + t1777 + t1778 - t1781 + t1782 + t1783 + t1784 + t1786 + t1787 + t1789 + t1790 + t1791;
    t1922 = t1898 * t415;
    t1923 = t1877 * t415;
    t1924 = t1892 * t415;
    t1925 = t1646 * t415;
    t1926 = t1649 * t415;
    t1927 = t1836 * t415;
    t1928 = t1698 * t1834;
    t1929 = t1206 * t123;
    t1930 = t36 * t191;
    t1932 = t1698 * t1884;
    t1934 = t1850 * t633;
    t1935 = t2 * t550;
    t1936 = t1708 * t1935;
    t1937 = t1860 * t633;
    t1938 = -t1793 + t1922 + t1923 + t1924 + t1925 + t1926 + t1927 + t1796 + t1799 + t1802 + t1928 + t1929 + 0.2e1 * t1930 - 0.2e1 * t1932 + t1934 + t1936 + t1937;
    t1939 = t1705 * t1834;
    t1940 = t288 * t123;
    t1941 = t42 * t191;
    t1943 = t1705 * t1884;
    t1945 = t1711 * t1935;
    t1946 = t1902 * t1844;
    t1947 = t679 * t1844;
    t1948 = t1939 + t1940 + 0.2e1 * t1941 - 0.2e1 * t1943 + t1945 + t1946 + t1947 + t1805 + t1808 + t1811 + t1814 + t1817 - t1819 - t1821 + t1823 + t1825 + t1828;
    t1952 = t1446 * (t1859 + t1879 + t1915 + t1916 + t1919 + t1920 + t1938 + t1948);
    SC_eval(5) = 0.12e2 * t1688 * t1562 + 0.12e2 * t1604 * t1446 * (t1731 + t1760 + t1785 + t1829) - 0.12e2 * t1685 * t1952;
    t1976 = -0.24e2 * t1183 * t256 + 0.2e1 * t1634 * t850 - 0.2e1 * t248 * t695 + 0.24e2 * t288 * t632 - 0.24e2 * t1837 + 0.48e2 * t1838 + 0.24e2 * t1839 + 0.48e2 * t1840 + 0.24e2 * t1841 + 0.48e2 * t1842 + 0.24e2 * t1843 + 0.24e2 * t1846 + 0.24e2 * t1848 + 0.12e2 * t551;
    t1997 = 0.24e2 * t105 * t632 + 0.24e2 * t231 * t632 + 0.24e2 * t234 * t632 + 0.2e1 * t240 * t632 + 0.24e2 * t632 * t84 + 0.48e2 * t1849 - 0.24e2 * t1851 + 0.24e2 * t1852 + 0.24e2 * t1853 + 0.24e2 * t1855 + 0.24e2 * t1858 - 0.24e2 * t1861 + 0.24e2 * t1862 + 0.24e2 * t1865 + 0.24e2 * t1866;
    t2015 = 0.2e1 * t101 * t632 - 0.48e2 * t1691 + 0.24e2 * t1695 + 0.24e2 * t1699 + 0.24e2 * t1703 + 0.24e2 * t1706 + 0.24e2 * t1709 + 0.24e2 * t1712 - 0.24e2 * t1867 + 0.48e2 * t1868 + 0.24e2 * t1870 + 0.72e2 * t1871 + 0.48e2 * t1875 - 0.24e2 * t1878 + 0.24e2 * t1882;
    t2035 = 0.2e1 * t110 * t29 + 0.24e2 * t110 * t30 + 0.24e2 * t110 * t34 + 0.24e2 * t110 * t46 + 0.24e2 * t1883 - 0.48e2 * t1886 - 0.48e2 * t1888 + 0.96e2 * t1890 - 0.24e2 * t1893 - 0.24e2 * t1894 + 0.48e2 * t1895 + 0.24e2 * t1897 - 0.24e2 * t1899 + 0.72e2 * t1900 + 0.48e2 * t1904;
    t2058 = 0.2e1 * t110 * t40 + 0.24e2 * t110 * t49 + 0.24e2 * t110 * t55 + 0.24e2 * t110 * t59 + 0.24e2 * t216 * t228 + 0.24e2 * t216 * t92 + 0.48e2 * t1716 + 0.12e2 * t1719 + 0.12e2 * t1721 + 0.12e2 * t1723 + 0.12e2 * t1725 + 0.48e2 * t1907 + 0.48e2 * t1910 + 0.96e2 * t1913;
    t2076 = 0.12e2 * t1421 * t582 + 0.12e2 * t21 * t597 + 0.12e2 * t1033 + 0.12e2 * t1102 + 0.12e2 * t1726 + 0.12e2 * t1727 + 0.12e2 * t1728 + 0.12e2 * t1729 + 0.12e2 * t1730 + 0.12e2 * t1732 + 0.12e2 * t1733 + 0.12e2 * t1734 + 0.12e2 * t1735 + 0.12e2 * t1736 + t913;
    t2103 = 0.12e2 * t10 * t597 + 0.12e2 * t1426 * t256 + 0.12e2 * t1429 * t256 + 0.12e2 * t1435 * t53 - 0.24e2 * t149 * t298 + 0.12e2 * t15 * t594 - 0.24e2 * t156 * t42 + t248 * t6 + t248 * t602 + t27 * t594 + 0.12e2 * t32 * t594 + 0.12e2 * t565 * t597 + 0.12e2 * t594 * t9 + 0.12e2 * t1042 + 0.12e2 * t1072;
    t2132 = -0.24e2 * t1045 * t149 - 0.24e2 * t1064 * t149 + 0.24e2 * t1086 * t645 - 0.24e2 * t156 * t36 + 0.24e2 * t261 * t645 + 0.12e2 * t261 * t775 + 0.12e2 * t261 * t779 + 0.12e2 * t270 * t6 + 0.12e2 * t270 * t602 + 0.12e2 * t522 * t6 + 0.12e2 * t522 * t602 + t526 * t6 + t526 * t602 + 0.12e2 * t530 * t6 + 0.12e2 * t530 * t602;
    t2166 = -0.24e2 * t357 * t52 * t666 - 0.24e2 * t52 * t57 * t666 + 0.24e2 * t1206 * t632 - 0.24e2 * t1551 * t666 + 0.2e1 * t1617 * t850 - 0.24e2 * t1690 * t261 - 0.24e2 * t270 * t695 + 0.24e2 * t278 * t645 + 0.12e2 * t411 * t6 + 0.12e2 * t411 * t602 - 0.24e2 * t411 * t695 - 0.24e2 * t522 * t695 - 0.2e1 * t526 * t695 - 0.24e2 * t530 * t695;
    t2182 = -0.12e2 * t1737 - 0.12e2 * t1739 + 0.24e2 * t1740 + 0.12e2 * t1742 + 0.12e2 * t1743 + 0.12e2 * t1744 + 0.12e2 * t1745 + 0.24e2 * t1746 + 0.24e2 * t1748 + 0.12e2 * t1750 - 0.24e2 * t1752 - 0.24e2 * t1756 - 0.12e2 * t1758 - 0.12e2 * t1759 + 0.24e2 * t1762;
    t2184 = t1765 + t12 + t24 + t1766 + t1767 + t1768 + t1769 + t1770 + t1771 + t1772 + t1773 + t1774 + t1775 + t1777 + t1778;
    t2201 = -0.24e2 * t1780 + 0.12e2 * t1782 + 0.12e2 * t1783 + 0.12e2 * t1784 + 0.12e2 * t1786 + 0.12e2 * t1787 + 0.12e2 * t1789 + 0.12e2 * t1790 + 0.12e2 * t1791 - 0.24e2 * t1792 + 0.24e2 * t1922 + 0.24e2 * t1923 + 0.24e2 * t1924 + 0.24e2 * t1925 + 0.24e2 * t1926;
    t2232 = 0.12e2 * t11 * t602 + 0.12e2 * t1162 * t1275 + 0.12e2 * t1162 * t1341 + 0.12e2 * t1345 * t1347 + 0.12e2 * t1345 * t54 - 0.12e2 * t149 * t559 - 0.12e2 * t149 * t569 + 0.24e2 * t16 * t597 + 0.24e2 * t16 * t612 + 0.24e2 * t195 * t612 + 0.12e2 * t246 * t562 + t28 * t597 + 0.13e2 * t28 * t612 + 0.13e2 * t357 * t612 + 0.24e2 * t1927;
    t2258 = t1110 * t1162 + 0.12e2 * t1345 * t255 - 0.12e2 * t149 * t41 - 0.12e2 * t149 * t579 + 0.24e2 * t195 * t597 + 0.12e2 * t23 * t602 + t246 * t38 + 0.12e2 * t246 * t44 + 0.12e2 * t246 * t572 + t357 * t597 + t57 * t597 + 0.13e2 * t57 * t612 + t579 * t645 + 0.12e2 * t1087 + 0.12e2 * t1123;
    t2278 = 0.12e2 * t246 * t552 + 0.24e2 * t33 * t597 + 0.24e2 * t33 * t612 + 0.24e2 * t1795 + 0.24e2 * t1798 + 0.48e2 * t1801 + 0.24e2 * t1928 + 0.48e2 * t1929 + 0.48e2 * t1930 - 0.48e2 * t1932 + 0.24e2 * t1934 + 0.24e2 * t1936 + 0.24e2 * t1937 + 0.24e2 * t1939 + 0.48e2 * t1940;
    t2294 = 0.48e2 * t1941 - 0.48e2 * t1943 + 0.24e2 * t1945 + 0.24e2 * t1946 + 0.24e2 * t1947 + 0.24e2 * t1804 + 0.24e2 * t1807 + 0.24e2 * t1810 + 0.24e2 * t1813 + 0.24e2 * t1816 - 0.24e2 * t1818 - 0.24e2 * t1820 + 0.24e2 * t1822 + 0.24e2 * t1824 + 0.24e2 * t1827;
    t2209 = t1976 + t1997 + t2015 + t2035 + t2058 + t2076 + t2103 + t2132 + t2166 + t2182 + 0.12e2 * t2184 + t2201 + t2232 + t2258 + t2278 + t2294;
    SC_eval(6) = t1446 * t1685 * t2209 - 0.12e2 * t1604 * t1952 - t1658 * t1688;
    SC_state_dot(1:6) = SC_eval(1:6);
end

== matlab function A2_2_Inverses_Pendel_PR/SimCodeGen_mfun_model/output_fun ==
  data: SC_state input size=[6]; SC_output_0 output size=[6]; SC_param_0 parameter size=[20]
function SC_output_0  = y_fun(SC_state, SC_param_0)
    SC_output_0 = zeros(6,1);
    SC_state_x_0 = SC_state(1:6);
    SC_output_0(1) = SC_state_x_0(1);
    SC_output_0(2) = SC_state_x_0(2);
    SC_output_0(3) = SC_state_x_0(3);
    SC_output_0(4) = SC_state_x_0(4);
    SC_output_0(5) = SC_state_x_0(5);
    SC_output_0(6) = SC_state_x_0(6);
end
